simulink model "Function_Teste"  (R2018a)
settings: Solver=VariableStepAuto  StartTime=0.0  StopTime=10.0  RelTol=1e-3
settings Model: Creator=marco  LastModifiedBy=marco

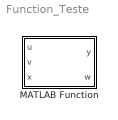
== system Function_Teste ==
  MATLAB Function : MATLAB Function  TreatAsAtomicUnit=on

== matlab function Function_Teste/MATLAB Function ==
  data: u input; y output; v input; x input; w output
function [y,w] = fcn(u,v,x)

y = u;
